simulink model "SPGF_FSK_0000_R2019b"  (R2019b)
settings: Solver=ode3  SolverName=ode4  StartTime=0.0  StopTime=1.4  FixedStep=50e-6/50  RelTol=1e-3  EnableMultiTasking=on
undefined symbols (not defined in the file): D11, Delta
libraries: powerlib x2544, powerlib_meascontrol x204, simulink x24
(part 32 of 33)

== system SPGF_FSK_0000_R2019b/W12/Q/breaker ==
  Fault A2 : Constant  Value=InitialStatus(3)
  Fault A3 : Constant  Value=InitialStatus(2)
  Fault A4 : Constant  Value=InitialStatus(1)
  Fault C1 : Constant  Value=SwitchC
  Fault C2 : Constant  Value=SwitchB
  Fault C3 : Constant  Value=SwitchA
  Ideal Switch A : powerlib/Power Electronics/Ideal Switch  Ron=BreakerResistance  Lon=0  IC=InitialStatus(1)  Rs=SnubberResistance  Cs=SnubberCapacitance  Measurements=off
  Ideal Switch B : powerlib/Power Electronics/Ideal Switch  Ron=BreakerResistance  Lon=0  IC=InitialStatus(2)  Rs=SnubberResistance  Cs=SnubberCapacitance  Measurements=off
  Ideal Switch C : powerlib/Power Electronics/Ideal Switch  Ron=BreakerResistance  Lon=0  IC=InitialStatus(3)  Rs=SnubberResistance  Cs=SnubberCapacitance  Measurements=off
  Stair Generator A : powerlib_meascontrol/Pulse & Signal Generators/Stair Generator  t=SwitchTimesA  e=SwitchStatusA  Ts=0
  Stair Generator B : powerlib_meascontrol/Pulse & Signal Generators/Stair Generator  t=SwitchTimesB  e=SwitchStatusB  Ts=0
  Stair Generator C : powerlib_meascontrol/Pulse & Signal Generators/Stair Generator  t=SwitchTimesB  e=SwitchStatusB  Ts=0
  Switch2 : Switch  Criteria=u2 > Threshold  Threshold=0.5
  Switch3 : Switch  Criteria=u2 > Threshold  Threshold=0.5
  Switch4 : Switch  Criteria=u2 > Threshold  Threshold=0.5
  A : PMIOPort  Side=Left
  B : PMIOPort  Port=2  Side=Left
  C : PMIOPort  Port=3  Side=Left
  a : PMIOPort  Port=4  Side=Right
  b : PMIOPort  Port=5  Side=Right
  c : PMIOPort  Port=6  Side=Right
  wires:
  Switch2/1 -> Ideal Switch C/1
  Fault A2/1 -> Switch2/3
  Fault C1/1 -> Switch2/2
  Switch3/1 -> Ideal Switch B/1
  Fault A3/1 -> Switch3/3
  Fault C2/1 -> Switch3/2
  Fault A4/1 -> Switch4/3
  Fault C3/1 -> Switch4/2
  Switch4/1 -> Ideal Switch A/1
  Stair Generator B/1 -> Switch3/1
  Stair Generator A/1 -> Switch4/1
  Stair Generator C/1 -> Switch2/1
  connections:
  Ideal Switch B/LConn1 -- B/RConn1
  Ideal Switch A/LConn1 -- A/RConn1
  Ideal Switch C/LConn1 -- C/RConn1
  Ideal Switch A/RConn1 -- a/RConn1
  b/RConn1 -- Ideal Switch B/RConn1
  c/RConn1 -- Ideal Switch C/RConn1

== system SPGF_FSK_0000_R2019b/W12/Q/meas ==
  Add : Sum  Inputs=+++
  GainI : Gain
  GainI0 : Gain
  I A: : powerlib/Measurements/Current Measurement  PhasorSimulation=off  OutputType=Complex  PSBequivalent=0
  I B: : powerlib/Measurements/Current Measurement  PhasorSimulation=off  OutputType=Complex  PSBequivalent=0
  I C: : powerlib/Measurements/Current Measurement  PhasorSimulation=off  OutputType=Complex  PSBequivalent=0
  Mux : Mux  Inputs=3
  A : PMIOPort  Side=Left
  B : PMIOPort  Port=2  Side=Left
  C : PMIOPort  Port=3  Side=Left
  a : PMIOPort  Port=4  Side=Right
  b : PMIOPort  Port=5  Side=Right
  c : PMIOPort  Port=6  Side=Right
  tag scope: CT3I0_W12=global, CTIabc_W12=global
  wires:
  I A:/1 -> Mux/1, Add/1
  I B:/1 -> Mux/2, Add/2
  I C:/1 -> Mux/3, Add/3
  Add/1 -> GainI0/1
  GainI0/1 -> [CT3I0_W12]
  Mux/1 -> GainI/1
  GainI/1 -> [CTIabc_W12]
  connections:
  I C:/RConn1 -- c/RConn1
  I B:/RConn1 -- b/RConn1
  a/RConn1 -- I A:/RConn1
  I A:/LConn1 -- A/RConn1
  I C:/LConn1 -- C/RConn1
  I B:/LConn1 -- B/RConn1

== system SPGF_FSK_0000_R2019b/W12/Q/shunt ==
  A : PMIOPort  Side=Left
  B : PMIOPort  Port=2  Side=Left
  C : PMIOPort  Port=3  Side=Left
  a : PMIOPort  Port=4  Side=Right
  b : PMIOPort  Port=5  Side=Right
  c : PMIOPort  Port=6  Side=Right
  connections:
  C/RConn1 -- c/RConn1
  B/RConn1 -- b/RConn1
  A/RConn1 -- a/RConn1

== system SPGF_FSK_0000_R2019b/W13/Q/breaker ==
  Fault A2 : Constant  Value=InitialStatus(3)
  Fault A3 : Constant  Value=InitialStatus(2)
  Fault A4 : Constant  Value=InitialStatus(1)
  Fault C1 : Constant  Value=SwitchC
  Fault C2 : Constant  Value=SwitchB
  Fault C3 : Constant  Value=SwitchA
  Ideal Switch A : powerlib/Power Electronics/Ideal Switch  Ron=BreakerResistance  Lon=0  IC=InitialStatus(1)  Rs=SnubberResistance  Cs=SnubberCapacitance  Measurements=off
  Ideal Switch B : powerlib/Power Electronics/Ideal Switch  Ron=BreakerResistance  Lon=0  IC=InitialStatus(2)  Rs=SnubberResistance  Cs=SnubberCapacitance  Measurements=off
  Ideal Switch C : powerlib/Power Electronics/Ideal Switch  Ron=BreakerResistance  Lon=0  IC=InitialStatus(3)  Rs=SnubberResistance  Cs=SnubberCapacitance  Measurements=off
  Stair Generator A : powerlib_meascontrol/Pulse & Signal Generators/Stair Generator  t=SwitchTimesA  e=SwitchStatusA  Ts=0
  Stair Generator B : powerlib_meascontrol/Pulse & Signal Generators/Stair Generator  t=SwitchTimesB  e=SwitchStatusB  Ts=0
  Stair Generator C : powerlib_meascontrol/Pulse & Signal Generators/Stair Generator  t=SwitchTimesB  e=SwitchStatusB  Ts=0
  Switch2 : Switch  Criteria=u2 > Threshold  Threshold=0.5
  Switch3 : Switch  Criteria=u2 > Threshold  Threshold=0.5
  Switch4 : Switch  Criteria=u2 > Threshold  Threshold=0.5
  A : PMIOPort  Side=Left
  B : PMIOPort  Port=2  Side=Left
  C : PMIOPort  Port=3  Side=Left
  a : PMIOPort  Port=4  Side=Right
  b : PMIOPort  Port=5  Side=Right
  c : PMIOPort  Port=6  Side=Right
  wires:
  Switch2/1 -> Ideal Switch C/1
  Fault A2/1 -> Switch2/3
  Fault C1/1 -> Switch2/2
  Switch3/1 -> Ideal Switch B/1
  Fault A3/1 -> Switch3/3
  Fault C2/1 -> Switch3/2
  Fault A4/1 -> Switch4/3
  Fault C3/1 -> Switch4/2
  Switch4/1 -> Ideal Switch A/1
  Stair Generator B/1 -> Switch3/1
  Stair Generator A/1 -> Switch4/1
  Stair Generator C/1 -> Switch2/1
  connections:
  Ideal Switch B/LConn1 -- B/RConn1
  Ideal Switch A/LConn1 -- A/RConn1
  Ideal Switch C/LConn1 -- C/RConn1
  Ideal Switch A/RConn1 -- a/RConn1
  b/RConn1 -- Ideal Switch B/RConn1
  c/RConn1 -- Ideal Switch C/RConn1

== system SPGF_FSK_0000_R2019b/W13/Q/meas ==
  Add : Sum  Inputs=+++
  GainI : Gain
  GainI0 : Gain
  I A: : powerlib/Measurements/Current Measurement  PhasorSimulation=off  OutputType=Complex  PSBequivalent=0
  I B: : powerlib/Measurements/Current Measurement  PhasorSimulation=off  OutputType=Complex  PSBequivalent=0
  I C: : powerlib/Measurements/Current Measurement  PhasorSimulation=off  OutputType=Complex  PSBequivalent=0
  Mux : Mux  Inputs=3
  A : PMIOPort  Side=Left
  B : PMIOPort  Port=2  Side=Left
  C : PMIOPort  Port=3  Side=Left
  a : PMIOPort  Port=4  Side=Right
  b : PMIOPort  Port=5  Side=Right
  c : PMIOPort  Port=6  Side=Right
  tag scope: CT3I0_W13=global, CTIabc_W13=global
  wires:
  I A:/1 -> Mux/1, Add/1
  I B:/1 -> Mux/2, Add/2
  I C:/1 -> Mux/3, Add/3
  Add/1 -> GainI0/1
  GainI0/1 -> [CT3I0_W13]
  Mux/1 -> GainI/1
  GainI/1 -> [CTIabc_W13]
  connections:
  I C:/RConn1 -- c/RConn1
  I B:/RConn1 -- b/RConn1
  a/RConn1 -- I A:/RConn1
  I A:/LConn1 -- A/RConn1
  I C:/LConn1 -- C/RConn1
  I B:/LConn1 -- B/RConn1

== system SPGF_FSK_0000_R2019b/W13/Q/shunt ==
  A : PMIOPort  Side=Left
  B : PMIOPort  Port=2  Side=Left
  C : PMIOPort  Port=3  Side=Left
  a : PMIOPort  Port=4  Side=Right
  b : PMIOPort  Port=5  Side=Right
  c : PMIOPort  Port=6  Side=Right
  connections:
  C/RConn1 -- c/RConn1
  B/RConn1 -- b/RConn1
  A/RConn1 -- a/RConn1

== system SPGF_FSK_0000_R2019b/W14/Q/breaker ==
  Fault A2 : Constant  Value=InitialStatus(3)
  Fault A3 : Constant  Value=InitialStatus(2)
  Fault A4 : Constant  Value=InitialStatus(1)
  Fault C1 : Constant  Value=SwitchC
  Fault C2 : Constant  Value=SwitchB
  Fault C3 : Constant  Value=SwitchA
  Ideal Switch A : powerlib/Power Electronics/Ideal Switch  Ron=BreakerResistance  Lon=0  IC=InitialStatus(1)  Rs=SnubberResistance  Cs=SnubberCapacitance  Measurements=off
  Ideal Switch B : powerlib/Power Electronics/Ideal Switch  Ron=BreakerResistance  Lon=0  IC=InitialStatus(2)  Rs=SnubberResistance  Cs=SnubberCapacitance  Measurements=off
  Ideal Switch C : powerlib/Power Electronics/Ideal Switch  Ron=BreakerResistance  Lon=0  IC=InitialStatus(3)  Rs=SnubberResistance  Cs=SnubberCapacitance  Measurements=off
  Stair Generator A : powerlib_meascontrol/Pulse & Signal Generators/Stair Generator  t=SwitchTimesA  e=SwitchStatusA  Ts=0
  Stair Generator B : powerlib_meascontrol/Pulse & Signal Generators/Stair Generator  t=SwitchTimesB  e=SwitchStatusB  Ts=0
  Stair Generator C : powerlib_meascontrol/Pulse & Signal Generators/Stair Generator  t=SwitchTimesB  e=SwitchStatusB  Ts=0
  Switch2 : Switch  Criteria=u2 > Threshold  Threshold=0.5
  Switch3 : Switch  Criteria=u2 > Threshold  Threshold=0.5
  Switch4 : Switch  Criteria=u2 > Threshold  Threshold=0.5
  A : PMIOPort  Side=Left
  B : PMIOPort  Port=2  Side=Left
  C : PMIOPort  Port=3  Side=Left
  a : PMIOPort  Port=4  Side=Right
  b : PMIOPort  Port=5  Side=Right
  c : PMIOPort  Port=6  Side=Right
  wires:
  Switch2/1 -> Ideal Switch C/1
  Fault A2/1 -> Switch2/3
  Fault C1/1 -> Switch2/2
  Switch3/1 -> Ideal Switch B/1
  Fault A3/1 -> Switch3/3
  Fault C2/1 -> Switch3/2
  Fault A4/1 -> Switch4/3
  Fault C3/1 -> Switch4/2
  Switch4/1 -> Ideal Switch A/1
  Stair Generator B/1 -> Switch3/1
  Stair Generator A/1 -> Switch4/1
  Stair Generator C/1 -> Switch2/1
  connections:
  Ideal Switch B/LConn1 -- B/RConn1
  Ideal Switch A/LConn1 -- A/RConn1
  Ideal Switch C/LConn1 -- C/RConn1
  Ideal Switch A/RConn1 -- a/RConn1
  b/RConn1 -- Ideal Switch B/RConn1
  c/RConn1 -- Ideal Switch C/RConn1

== system SPGF_FSK_0000_R2019b/W14/Q/meas ==
  Add : Sum  Inputs=+++
  GainI : Gain
  GainI0 : Gain
  I A: : powerlib/Measurements/Current Measurement  PhasorSimulation=off  OutputType=Complex  PSBequivalent=0
  I B: : powerlib/Measurements/Current Measurement  PhasorSimulation=off  OutputType=Complex  PSBequivalent=0
  I C: : powerlib/Measurements/Current Measurement  PhasorSimulation=off  OutputType=Complex  PSBequivalent=0
  Mux : Mux  Inputs=3
  A : PMIOPort  Side=Left
  B : PMIOPort  Port=2  Side=Left
  C : PMIOPort  Port=3  Side=Left
  a : PMIOPort  Port=4  Side=Right
  b : PMIOPort  Port=5  Side=Right
  c : PMIOPort  Port=6  Side=Right
  tag scope: CT3I0_W14=global, CTIabc_W14=global
  wires:
  I A:/1 -> Mux/1, Add/1
  I B:/1 -> Mux/2, Add/2
  I C:/1 -> Mux/3, Add/3
  Add/1 -> GainI0/1
  GainI0/1 -> [CT3I0_W14]
  Mux/1 -> GainI/1
  GainI/1 -> [CTIabc_W14]
  connections:
  I C:/RConn1 -- c/RConn1
  I B:/RConn1 -- b/RConn1
  a/RConn1 -- I A:/RConn1
  I A:/LConn1 -- A/RConn1
  I C:/LConn1 -- C/RConn1
  I B:/LConn1 -- B/RConn1

== system SPGF_FSK_0000_R2019b/W14/Q/shunt ==
  A : PMIOPort  Side=Left
  B : PMIOPort  Port=2  Side=Left
  C : PMIOPort  Port=3  Side=Left
  a : PMIOPort  Port=4  Side=Right
  b : PMIOPort  Port=5  Side=Right
  c : PMIOPort  Port=6  Side=Right
  connections:
  C/RConn1 -- c/RConn1
  B/RConn1 -- b/RConn1
  A/RConn1 -- a/RConn1

== system SPGF_FSK_0000_R2019b/W15/Q/breaker ==
  Fault A2 : Constant  Value=InitialStatus(3)
  Fault A3 : Constant  Value=InitialStatus(2)
  Fault A4 : Constant  Value=InitialStatus(1)
  Fault C1 : Constant  Value=SwitchC
  Fault C2 : Constant  Value=SwitchB
  Fault C3 : Constant  Value=SwitchA
  Ideal Switch A : powerlib/Power Electronics/Ideal Switch  Ron=BreakerResistance  Lon=0  IC=InitialStatus(1)  Rs=SnubberResistance  Cs=SnubberCapacitance  Measurements=off
  Ideal Switch B : powerlib/Power Electronics/Ideal Switch  Ron=BreakerResistance  Lon=0  IC=InitialStatus(2)  Rs=SnubberResistance  Cs=SnubberCapacitance  Measurements=off
  Ideal Switch C : powerlib/Power Electronics/Ideal Switch  Ron=BreakerResistance  Lon=0  IC=InitialStatus(3)  Rs=SnubberResistance  Cs=SnubberCapacitance  Measurements=off
  Stair Generator A : powerlib_meascontrol/Pulse & Signal Generators/Stair Generator  t=SwitchTimesA  e=SwitchStatusA  Ts=0
  Stair Generator B : powerlib_meascontrol/Pulse & Signal Generators/Stair Generator  t=SwitchTimesB  e=SwitchStatusB  Ts=0
  Stair Generator C : powerlib_meascontrol/Pulse & Signal Generators/Stair Generator  t=SwitchTimesB  e=SwitchStatusB  Ts=0
  Switch2 : Switch  Criteria=u2 > Threshold  Threshold=0.5
  Switch3 : Switch  Criteria=u2 > Threshold  Threshold=0.5
  Switch4 : Switch  Criteria=u2 > Threshold  Threshold=0.5
  A : PMIOPort  Side=Left
  B : PMIOPort  Port=2  Side=Left
  C : PMIOPort  Port=3  Side=Left
  a : PMIOPort  Port=4  Side=Right
  b : PMIOPort  Port=5  Side=Right
  c : PMIOPort  Port=6  Side=Right
  wires:
  Switch2/1 -> Ideal Switch C/1
  Fault A2/1 -> Switch2/3
  Fault C1/1 -> Switch2/2
  Switch3/1 -> Ideal Switch B/1
  Fault A3/1 -> Switch3/3
  Fault C2/1 -> Switch3/2
  Fault A4/1 -> Switch4/3
  Fault C3/1 -> Switch4/2
  Switch4/1 -> Ideal Switch A/1
  Stair Generator B/1 -> Switch3/1
  Stair Generator A/1 -> Switch4/1
  Stair Generator C/1 -> Switch2/1
  connections:
  Ideal Switch B/LConn1 -- B/RConn1
  Ideal Switch A/LConn1 -- A/RConn1
  Ideal Switch C/LConn1 -- C/RConn1
  Ideal Switch A/RConn1 -- a/RConn1
  b/RConn1 -- Ideal Switch B/RConn1
  c/RConn1 -- Ideal Switch C/RConn1

== system SPGF_FSK_0000_R2019b/W15/Q/meas ==
  Add : Sum  Inputs=+++
  GainI : Gain
  GainI0 : Gain
  I A: : powerlib/Measurements/Current Measurement  PhasorSimulation=off  OutputType=Complex  PSBequivalent=0
  I B: : powerlib/Measurements/Current Measurement  PhasorSimulation=off  OutputType=Complex  PSBequivalent=0
  I C: : powerlib/Measurements/Current Measurement  PhasorSimulation=off  OutputType=Complex  PSBequivalent=0
  Mux : Mux  Inputs=3
  A : PMIOPort  Side=Left
  B : PMIOPort  Port=2  Side=Left
  C : PMIOPort  Port=3  Side=Left
  a : PMIOPort  Port=4  Side=Right
  b : PMIOPort  Port=5  Side=Right
  c : PMIOPort  Port=6  Side=Right
  tag scope: CT3I0_W15=global, CTIabc_W15=global
  wires:
  I A:/1 -> Mux/1, Add/1
  I B:/1 -> Mux/2, Add/2
  I C:/1 -> Mux/3, Add/3
  Add/1 -> GainI0/1
  GainI0/1 -> [CT3I0_W15]
  Mux/1 -> GainI/1
  GainI/1 -> [CTIabc_W15]
  connections:
  I C:/RConn1 -- c/RConn1
  I B:/RConn1 -- b/RConn1
  a/RConn1 -- I A:/RConn1
  I A:/LConn1 -- A/RConn1
  I C:/LConn1 -- C/RConn1
  I B:/LConn1 -- B/RConn1

== system SPGF_FSK_0000_R2019b/W15/Q/shunt ==
  A : PMIOPort  Side=Left
  B : PMIOPort  Port=2  Side=Left
  C : PMIOPort  Port=3  Side=Left
  a : PMIOPort  Port=4  Side=Right
  b : PMIOPort  Port=5  Side=Right
  c : PMIOPort  Port=6  Side=Right
  connections:
  C/RConn1 -- c/RConn1
  B/RConn1 -- b/RConn1
  A/RConn1 -- a/RConn1

== system SPGF_FSK_0000_R2019b/W21/Q/breaker ==
  Fault A2 : Constant  Value=InitialStatus(3)
  Fault A3 : Constant  Value=InitialStatus(2)
  Fault A4 : Constant  Value=InitialStatus(1)
  Fault C1 : Constant  Value=SwitchC
  Fault C2 : Constant  Value=SwitchB
  Fault C3 : Constant  Value=SwitchA
  Ideal Switch A : powerlib/Power Electronics/Ideal Switch  Ron=BreakerResistance  Lon=0  IC=InitialStatus(1)  Rs=SnubberResistance  Cs=SnubberCapacitance  Measurements=off
  Ideal Switch B : powerlib/Power Electronics/Ideal Switch  Ron=BreakerResistance  Lon=0  IC=InitialStatus(2)  Rs=SnubberResistance  Cs=SnubberCapacitance  Measurements=off
  Ideal Switch C : powerlib/Power Electronics/Ideal Switch  Ron=BreakerResistance  Lon=0  IC=InitialStatus(3)  Rs=SnubberResistance  Cs=SnubberCapacitance  Measurements=off
  Stair Generator A : powerlib_meascontrol/Pulse & Signal Generators/Stair Generator  t=SwitchTimesA  e=SwitchStatusA  Ts=0
  Stair Generator B : powerlib_meascontrol/Pulse & Signal Generators/Stair Generator  t=SwitchTimesB  e=SwitchStatusB  Ts=0
  Stair Generator C : powerlib_meascontrol/Pulse & Signal Generators/Stair Generator  t=SwitchTimesC  e=SwitchStatusC  Ts=0
  Switch2 : Switch  Criteria=u2 > Threshold  Threshold=0.5
  Switch3 : Switch  Criteria=u2 > Threshold  Threshold=0.5
  Switch4 : Switch  Criteria=u2 > Threshold  Threshold=0.5
  A : PMIOPort  Side=Left
  B : PMIOPort  Port=2  Side=Left
  C : PMIOPort  Port=3  Side=Left
  a : PMIOPort  Port=4  Side=Right
  b : PMIOPort  Port=5  Side=Right
  c : PMIOPort  Port=6  Side=Right
  wires:
  Switch2/1 -> Ideal Switch C/1
  Fault A2/1 -> Switch2/3
  Fault C1/1 -> Switch2/2
  Switch3/1 -> Ideal Switch B/1
  Fault A3/1 -> Switch3/3
  Fault C2/1 -> Switch3/2
  Fault A4/1 -> Switch4/3
  Fault C3/1 -> Switch4/2
  Switch4/1 -> Ideal Switch A/1
  Stair Generator B/1 -> Switch3/1
  Stair Generator A/1 -> Switch4/1
  Stair Generator C/1 -> Switch2/1
  connections:
  Ideal Switch B/LConn1 -- B/RConn1
  Ideal Switch A/LConn1 -- A/RConn1
  Ideal Switch C/LConn1 -- C/RConn1
  Ideal Switch A/RConn1 -- a/RConn1
  b/RConn1 -- Ideal Switch B/RConn1
  c/RConn1 -- Ideal Switch C/RConn1

== system SPGF_FSK_0000_R2019b/W21/Q/meas ==
  Add : Sum  Inputs=+++
  GainI : Gain
  GainI0 : Gain
  I A: : powerlib/Measurements/Current Measurement  PhasorSimulation=off  OutputType=Complex  PSBequivalent=0
  I B: : powerlib/Measurements/Current Measurement  PhasorSimulation=off  OutputType=Complex  PSBequivalent=0
  I C: : powerlib/Measurements/Current Measurement  PhasorSimulation=off  OutputType=Complex  PSBequivalent=0
  Mux : Mux  Inputs=3
  A : PMIOPort  Side=Left
  B : PMIOPort  Port=2  Side=Left
  C : PMIOPort  Port=3  Side=Left
  a : PMIOPort  Port=4  Side=Right
  b : PMIOPort  Port=5  Side=Right
  c : PMIOPort  Port=6  Side=Right
  tag scope: CT3I0_W21=global, CTIabc_W21=global
  wires:
  I A:/1 -> Mux/1, Add/1
  I B:/1 -> Mux/2, Add/2
  I C:/1 -> Mux/3, Add/3
  Add/1 -> GainI0/1
  GainI0/1 -> [CT3I0_W21]
  Mux/1 -> GainI/1
  GainI/1 -> [CTIabc_W21]
  connections:
  I C:/RConn1 -- c/RConn1
  I B:/RConn1 -- b/RConn1
  a/RConn1 -- I A:/RConn1
  I A:/LConn1 -- A/RConn1
  I C:/LConn1 -- C/RConn1
  I B:/LConn1 -- B/RConn1

== system SPGF_FSK_0000_R2019b/W21/Q/shunt ==
  A : PMIOPort  Side=Left
  B : PMIOPort  Port=2  Side=Left
  C : PMIOPort  Port=3  Side=Left
  a : PMIOPort  Port=4  Side=Right
  b : PMIOPort  Port=5  Side=Right
  c : PMIOPort  Port=6  Side=Right
  connections:
  C/RConn1 -- c/RConn1
  B/RConn1 -- b/RConn1
  A/RConn1 -- a/RConn1

== system SPGF_FSK_0000_R2019b/W22/Q/breaker ==
  Fault A2 : Constant  Value=InitialStatus(3)
  Fault A3 : Constant  Value=InitialStatus(2)
  Fault A4 : Constant  Value=InitialStatus(1)
  Fault C1 : Constant  Value=SwitchC
  Fault C2 : Constant  Value=SwitchB
  Fault C3 : Constant  Value=SwitchA
  Ideal Switch A : powerlib/Power Electronics/Ideal Switch  Ron=BreakerResistance  Lon=0  IC=InitialStatus(1)  Rs=SnubberResistance  Cs=SnubberCapacitance  Measurements=off
  Ideal Switch B : powerlib/Power Electronics/Ideal Switch  Ron=BreakerResistance  Lon=0  IC=InitialStatus(2)  Rs=SnubberResistance  Cs=SnubberCapacitance  Measurements=off
  Ideal Switch C : powerlib/Power Electronics/Ideal Switch  Ron=BreakerResistance  Lon=0  IC=InitialStatus(3)  Rs=SnubberResistance  Cs=SnubberCapacitance  Measurements=off
  Stair Generator A : powerlib_meascontrol/Pulse & Signal Generators/Stair Generator  t=SwitchTimesA  e=SwitchStatusA  Ts=0
  Stair Generator B : powerlib_meascontrol/Pulse & Signal Generators/Stair Generator  t=SwitchTimesB  e=SwitchStatusB  Ts=0
  Stair Generator C : powerlib_meascontrol/Pulse & Signal Generators/Stair Generator  t=SwitchTimesB  e=SwitchStatusB  Ts=0
  Switch2 : Switch  Criteria=u2 > Threshold  Threshold=0.5
  Switch3 : Switch  Criteria=u2 > Threshold  Threshold=0.5
  Switch4 : Switch  Criteria=u2 > Threshold  Threshold=0.5
  A : PMIOPort  Side=Left
  B : PMIOPort  Port=2  Side=Left
  C : PMIOPort  Port=3  Side=Left
  a : PMIOPort  Port=4  Side=Right
  b : PMIOPort  Port=5  Side=Right
  c : PMIOPort  Port=6  Side=Right
  wires:
  Switch2/1 -> Ideal Switch C/1
  Fault A2/1 -> Switch2/3
  Fault C1/1 -> Switch2/2
  Switch3/1 -> Ideal Switch B/1
  Fault A3/1 -> Switch3/3
  Fault C2/1 -> Switch3/2
  Fault A4/1 -> Switch4/3
  Fault C3/1 -> Switch4/2
  Switch4/1 -> Ideal Switch A/1
  Stair Generator B/1 -> Switch3/1
  Stair Generator A/1 -> Switch4/1
  Stair Generator C/1 -> Switch2/1
  connections:
  Ideal Switch B/LConn1 -- B/RConn1
  Ideal Switch A/LConn1 -- A/RConn1
  Ideal Switch C/LConn1 -- C/RConn1
  Ideal Switch A/RConn1 -- a/RConn1
  b/RConn1 -- Ideal Switch B/RConn1
  c/RConn1 -- Ideal Switch C/RConn1

== system SPGF_FSK_0000_R2019b/W22/Q/meas ==
  Add : Sum  Inputs=+++
  GainI : Gain
  GainI0 : Gain
  I A: : powerlib/Measurements/Current Measurement  PhasorSimulation=off  OutputType=Complex  PSBequivalent=0
  I B: : powerlib/Measurements/Current Measurement  PhasorSimulation=off  OutputType=Complex  PSBequivalent=0
  I C: : powerlib/Measurements/Current Measurement  PhasorSimulation=off  OutputType=Complex  PSBequivalent=0
  Mux : Mux  Inputs=3
  A : PMIOPort  Side=Left
  B : PMIOPort  Port=2  Side=Left
  C : PMIOPort  Port=3  Side=Left
  a : PMIOPort  Port=4  Side=Right
  b : PMIOPort  Port=5  Side=Right
  c : PMIOPort  Port=6  Side=Right
  tag scope: CT3I0_W22=global, CTIabc_W22=global
  wires:
  I A:/1 -> Mux/1, Add/1
  I B:/1 -> Mux/2, Add/2
  I C:/1 -> Mux/3, Add/3
  Add/1 -> GainI0/1
  GainI0/1 -> [CT3I0_W22]
  Mux/1 -> GainI/1
  GainI/1 -> [CTIabc_W22]
  connections:
  I C:/RConn1 -- c/RConn1
  I B:/RConn1 -- b/RConn1
  a/RConn1 -- I A:/RConn1
  I A:/LConn1 -- A/RConn1
  I C:/LConn1 -- C/RConn1
  I B:/LConn1 -- B/RConn1

== system SPGF_FSK_0000_R2019b/W22/Q/shunt ==
  A : PMIOPort  Side=Left
  B : PMIOPort  Port=2  Side=Left
  C : PMIOPort  Port=3  Side=Left
  a : PMIOPort  Port=4  Side=Right
  b : PMIOPort  Port=5  Side=Right
  c : PMIOPort  Port=6  Side=Right
  connections:
  C/RConn1 -- c/RConn1
  B/RConn1 -- b/RConn1
  A/RConn1 -- a/RConn1

== system SPGF_FSK_0000_R2019b/W31/Q/breaker ==
  Fault A2 : Constant  Value=InitialStatus(3)
  Fault A3 : Constant  Value=InitialStatus(2)
  Fault A4 : Constant  Value=InitialStatus(1)
  Fault C1 : Constant  Value=SwitchC
  Fault C2 : Constant  Value=SwitchB
  Fault C3 : Constant  Value=SwitchA
  Ideal Switch A : powerlib/Power Electronics/Ideal Switch  Ron=BreakerResistance  Lon=0  IC=InitialStatus(1)  Rs=SnubberResistance  Cs=SnubberCapacitance  Measurements=off
  Ideal Switch B : powerlib/Power Electronics/Ideal Switch  Ron=BreakerResistance  Lon=0  IC=InitialStatus(2)  Rs=SnubberResistance  Cs=SnubberCapacitance  Measurements=off
  Ideal Switch C : powerlib/Power Electronics/Ideal Switch  Ron=BreakerResistance  Lon=0  IC=InitialStatus(3)  Rs=SnubberResistance  Cs=SnubberCapacitance  Measurements=off
  Stair Generator A : powerlib_meascontrol/Pulse & Signal Generators/Stair Generator  t=SwitchTimesA  e=SwitchStatusA  Ts=0
  Stair Generator B : powerlib_meascontrol/Pulse & Signal Generators/Stair Generator  t=SwitchTimesB  e=SwitchStatusB  Ts=0
  Stair Generator C : powerlib_meascontrol/Pulse & Signal Generators/Stair Generator  t=SwitchTimesC  e=SwitchStatusC  Ts=0
  Switch2 : Switch  Criteria=u2 > Threshold  Threshold=0.5
  Switch3 : Switch  Criteria=u2 > Threshold  Threshold=0.5
  Switch4 : Switch  Criteria=u2 > Threshold  Threshold=0.5
  A : PMIOPort  Side=Left
  B : PMIOPort  Port=2  Side=Left
  C : PMIOPort  Port=3  Side=Left
  a : PMIOPort  Port=4  Side=Right
  b : PMIOPort  Port=5  Side=Right
  c : PMIOPort  Port=6  Side=Right
  wires:
  Switch2/1 -> Ideal Switch C/1
  Fault A2/1 -> Switch2/3
  Fault C1/1 -> Switch2/2
  Switch3/1 -> Ideal Switch B/1
  Fault A3/1 -> Switch3/3
  Fault C2/1 -> Switch3/2
  Fault A4/1 -> Switch4/3
  Fault C3/1 -> Switch4/2
  Switch4/1 -> Ideal Switch A/1
  Stair Generator B/1 -> Switch3/1
  Stair Generator A/1 -> Switch4/1
  Stair Generator C/1 -> Switch2/1
  connections:
  Ideal Switch B/LConn1 -- B/RConn1
  Ideal Switch A/LConn1 -- A/RConn1
  Ideal Switch C/LConn1 -- C/RConn1
  Ideal Switch A/RConn1 -- a/RConn1
  b/RConn1 -- Ideal Switch B/RConn1
  c/RConn1 -- Ideal Switch C/RConn1

== system SPGF_FSK_0000_R2019b/W31/Q/meas ==
  Add : Sum  Inputs=+++
  GainI : Gain
  GainI0 : Gain
  I A: : powerlib/Measurements/Current Measurement  PhasorSimulation=off  OutputType=Complex  PSBequivalent=0
  I B: : powerlib/Measurements/Current Measurement  PhasorSimulation=off  OutputType=Complex  PSBequivalent=0
  I C: : powerlib/Measurements/Current Measurement  PhasorSimulation=off  OutputType=Complex  PSBequivalent=0
  Mux : Mux  Inputs=3
  A : PMIOPort  Side=Left
  B : PMIOPort  Port=2  Side=Left
  C : PMIOPort  Port=3  Side=Left
  a : PMIOPort  Port=4  Side=Right
  b : PMIOPort  Port=5  Side=Right
  c : PMIOPort  Port=6  Side=Right
  tag scope: CT3I0_W31=global, CTIabc_W31=global
  wires:
  I A:/1 -> Mux/1, Add/1
  I B:/1 -> Mux/2, Add/2
  I C:/1 -> Mux/3, Add/3
  Add/1 -> GainI0/1
  GainI0/1 -> [CT3I0_W31]
  Mux/1 -> GainI/1
  GainI/1 -> [CTIabc_W31]
  connections:
  I C:/RConn1 -- c/RConn1
  I B:/RConn1 -- b/RConn1
  a/RConn1 -- I A:/RConn1
  I A:/LConn1 -- A/RConn1
  I C:/LConn1 -- C/RConn1
  I B:/LConn1 -- B/RConn1

== system SPGF_FSK_0000_R2019b/W31/Q/shunt ==
  A : PMIOPort  Side=Left
  B : PMIOPort  Port=2  Side=Left
  C : PMIOPort  Port=3  Side=Left
  a : PMIOPort  Port=4  Side=Right
  b : PMIOPort  Port=5  Side=Right
  c : PMIOPort  Port=6  Side=Right
  connections:
  C/RConn1 -- c/RConn1
  B/RConn1 -- b/RConn1
  A/RConn1 -- a/RConn1

== system SPGF_FSK_0000_R2019b/W32/Q/breaker ==
  Fault A2 : Constant  Value=InitialStatus(3)
  Fault A3 : Constant  Value=InitialStatus(2)
  Fault A4 : Constant  Value=InitialStatus(1)
  Fault C1 : Constant  Value=SwitchC
  Fault C2 : Constant  Value=SwitchB
  Fault C3 : Constant  Value=SwitchA
  Ideal Switch A : powerlib/Power Electronics/Ideal Switch  Ron=BreakerResistance  Lon=0  IC=InitialStatus(1)  Rs=SnubberResistance  Cs=SnubberCapacitance  Measurements=off
  Ideal Switch B : powerlib/Power Electronics/Ideal Switch  Ron=BreakerResistance  Lon=0  IC=InitialStatus(2)  Rs=SnubberResistance  Cs=SnubberCapacitance  Measurements=off
  Ideal Switch C : powerlib/Power Electronics/Ideal Switch  Ron=BreakerResistance  Lon=0  IC=InitialStatus(3)  Rs=SnubberResistance  Cs=SnubberCapacitance  Measurements=off
  Stair Generator A : powerlib_meascontrol/Pulse & Signal Generators/Stair Generator  t=SwitchTimesA  e=SwitchStatusA  Ts=0
  Stair Generator B : powerlib_meascontrol/Pulse & Signal Generators/Stair Generator  t=SwitchTimesB  e=SwitchStatusB  Ts=0
  Stair Generator C : powerlib_meascontrol/Pulse & Signal Generators/Stair Generator  t=SwitchTimesB  e=SwitchStatusB  Ts=0
  Switch2 : Switch  Criteria=u2 > Threshold  Threshold=0.5
  Switch3 : Switch  Criteria=u2 > Threshold  Threshold=0.5
  Switch4 : Switch  Criteria=u2 > Threshold  Threshold=0.5
  A : PMIOPort  Side=Left
  B : PMIOPort  Port=2  Side=Left
  C : PMIOPort  Port=3  Side=Left
  a : PMIOPort  Port=4  Side=Right
  b : PMIOPort  Port=5  Side=Right
  c : PMIOPort  Port=6  Side=Right
  wires:
  Switch2/1 -> Ideal Switch C/1
  Fault A2/1 -> Switch2/3
  Fault C1/1 -> Switch2/2
  Switch3/1 -> Ideal Switch B/1
  Fault A3/1 -> Switch3/3
  Fault C2/1 -> Switch3/2
  Fault A4/1 -> Switch4/3
  Fault C3/1 -> Switch4/2
  Switch4/1 -> Ideal Switch A/1
  Stair Generator B/1 -> Switch3/1
  Stair Generator A/1 -> Switch4/1
  Stair Generator C/1 -> Switch2/1
  connections:
  Ideal Switch B/LConn1 -- B/RConn1
  Ideal Switch A/LConn1 -- A/RConn1
  Ideal Switch C/LConn1 -- C/RConn1
  Ideal Switch A/RConn1 -- a/RConn1
  b/RConn1 -- Ideal Switch B/RConn1
  c/RConn1 -- Ideal Switch C/RConn1

== system SPGF_FSK_0000_R2019b/W32/Q/meas ==
  Add : Sum  Inputs=+++
  GainI : Gain
  GainI0 : Gain
  I A: : powerlib/Measurements/Current Measurement  PhasorSimulation=off  OutputType=Complex  PSBequivalent=0
  I B: : powerlib/Measurements/Current Measurement  PhasorSimulation=off  OutputType=Complex  PSBequivalent=0
  I C: : powerlib/Measurements/Current Measurement  PhasorSimulation=off  OutputType=Complex  PSBequivalent=0
  Mux : Mux  Inputs=3
  A : PMIOPort  Side=Left
  B : PMIOPort  Port=2  Side=Left
  C : PMIOPort  Port=3  Side=Left
  a : PMIOPort  Port=4  Side=Right
  b : PMIOPort  Port=5  Side=Right
  c : PMIOPort  Port=6  Side=Right
  tag scope: CT3I0_W32=global, CTIabc_W32=global
  wires:
  I A:/1 -> Mux/1, Add/1
  I B:/1 -> Mux/2, Add/2
  I C:/1 -> Mux/3, Add/3
  Add/1 -> GainI0/1
  GainI0/1 -> [CT3I0_W32]
  Mux/1 -> GainI/1
  GainI/1 -> [CTIabc_W32]
  connections:
  I C:/RConn1 -- c/RConn1
  I B:/RConn1 -- b/RConn1
  a/RConn1 -- I A:/RConn1
  I A:/LConn1 -- A/RConn1
  I C:/LConn1 -- C/RConn1
  I B:/LConn1 -- B/RConn1

== system SPGF_FSK_0000_R2019b/W32/Q/shunt ==
  A : PMIOPort  Side=Left
  B : PMIOPort  Port=2  Side=Left
  C : PMIOPort  Port=3  Side=Left
  a : PMIOPort  Port=4  Side=Right
  b : PMIOPort  Port=5  Side=Right
  c : PMIOPort  Port=6  Side=Right
  connections:
  C/RConn1 -- c/RConn1
  B/RConn1 -- b/RConn1
  A/RConn1 -- a/RConn1

== system SPGF_FSK_0000_R2019b/W33/Q/breaker ==
  Fault A2 : Constant  Value=InitialStatus(3)
  Fault A3 : Constant  Value=InitialStatus(2)
  Fault A4 : Constant  Value=InitialStatus(1)
  Fault C1 : Constant  Value=SwitchC
  Fault C2 : Constant  Value=SwitchB
  Fault C3 : Constant  Value=SwitchA
  Ideal Switch A : powerlib/Power Electronics/Ideal Switch  Ron=BreakerResistance  Lon=0  IC=InitialStatus(1)  Rs=SnubberResistance  Cs=SnubberCapacitance  Measurements=off
  Ideal Switch B : powerlib/Power Electronics/Ideal Switch  Ron=BreakerResistance  Lon=0  IC=InitialStatus(2)  Rs=SnubberResistance  Cs=SnubberCapacitance  Measurements=off
  Ideal Switch C : powerlib/Power Electronics/Ideal Switch  Ron=BreakerResistance  Lon=0  IC=InitialStatus(3)  Rs=SnubberResistance  Cs=SnubberCapacitance  Measurements=off
  Stair Generator A : powerlib_meascontrol/Pulse & Signal Generators/Stair Generator  t=SwitchTimesA  e=SwitchStatusA  Ts=0
  Stair Generator B : powerlib_meascontrol/Pulse & Signal Generators/Stair Generator  t=SwitchTimesB  e=SwitchStatusB  Ts=0
  Stair Generator C : powerlib_meascontrol/Pulse & Signal Generators/Stair Generator  t=SwitchTimesB  e=SwitchStatusB  Ts=0
  Switch2 : Switch  Criteria=u2 > Threshold  Threshold=0.5
  Switch3 : Switch  Criteria=u2 > Threshold  Threshold=0.5
  Switch4 : Switch  Criteria=u2 > Threshold  Threshold=0.5
  A : PMIOPort  Side=Left
  B : PMIOPort  Port=2  Side=Left
  C : PMIOPort  Port=3  Side=Left
  a : PMIOPort  Port=4  Side=Right
  b : PMIOPort  Port=5  Side=Right
  c : PMIOPort  Port=6  Side=Right
  wires:
  Switch2/1 -> Ideal Switch C/1
  Fault A2/1 -> Switch2/3
  Fault C1/1 -> Switch2/2
  Switch3/1 -> Ideal Switch B/1
  Fault A3/1 -> Switch3/3
  Fault C2/1 -> Switch3/2
  Fault A4/1 -> Switch4/3
  Fault C3/1 -> Switch4/2
  Switch4/1 -> Ideal Switch A/1
  Stair Generator B/1 -> Switch3/1
  Stair Generator A/1 -> Switch4/1
  Stair Generator C/1 -> Switch2/1
  connections:
  Ideal Switch B/LConn1 -- B/RConn1
  Ideal Switch A/LConn1 -- A/RConn1
  Ideal Switch C/LConn1 -- C/RConn1
  Ideal Switch A/RConn1 -- a/RConn1
  b/RConn1 -- Ideal Switch B/RConn1
  c/RConn1 -- Ideal Switch C/RConn1

== system SPGF_FSK_0000_R2019b/W33/Q/meas ==
  Add : Sum  Inputs=+++
  GainI : Gain
  GainI0 : Gain
  I A: : powerlib/Measurements/Current Measurement  PhasorSimulation=off  OutputType=Complex  PSBequivalent=0
  I B: : powerlib/Measurements/Current Measurement  PhasorSimulation=off  OutputType=Complex  PSBequivalent=0
  I C: : powerlib/Measurements/Current Measurement  PhasorSimulation=off  OutputType=Complex  PSBequivalent=0
  Mux : Mux  Inputs=3
  A : PMIOPort  Side=Left
  B : PMIOPort  Port=2  Side=Left
  C : PMIOPort  Port=3  Side=Left
  a : PMIOPort  Port=4  Side=Right
  b : PMIOPort  Port=5  Side=Right
  c : PMIOPort  Port=6  Side=Right
  tag scope: CT3I0_W33=global, CTIabc_W33=global
  wires:
  I A:/1 -> Mux/1, Add/1
  I B:/1 -> Mux/2, Add/2
  I C:/1 -> Mux/3, Add/3
  Add/1 -> GainI0/1
  GainI0/1 -> [CT3I0_W33]
  Mux/1 -> GainI/1
  GainI/1 -> [CTIabc_W33]
  connections:
  I C:/RConn1 -- c/RConn1
  I B:/RConn1 -- b/RConn1
  a/RConn1 -- I A:/RConn1
  I A:/LConn1 -- A/RConn1
  I C:/LConn1 -- C/RConn1
  I B:/LConn1 -- B/RConn1

== system SPGF_FSK_0000_R2019b/W33/Q/shunt ==
  A : PMIOPort  Side=Left
  B : PMIOPort  Port=2  Side=Left
  C : PMIOPort  Port=3  Side=Left
  a : PMIOPort  Port=4  Side=Right
  b : PMIOPort  Port=5  Side=Right
  c : PMIOPort  Port=6  Side=Right
  connections:
  C/RConn1 -- c/RConn1
  B/RConn1 -- b/RConn1
  A/RConn1 -- a/RConn1

== system SPGF_FSK_0000_R2019b/W34/Q/breaker ==
  Fault A2 : Constant  Value=InitialStatus(3)
  Fault A3 : Constant  Value=InitialStatus(2)
  Fault A4 : Constant  Value=InitialStatus(1)
  Fault C1 : Constant  Value=SwitchC
  Fault C2 : Constant  Value=SwitchB
  Fault C3 : Constant  Value=SwitchA
  Ideal Switch A : powerlib/Power Electronics/Ideal Switch  Ron=BreakerResistance  Lon=0  IC=InitialStatus(1)  Rs=SnubberResistance  Cs=SnubberCapacitance  Measurements=off
  Ideal Switch B : powerlib/Power Electronics/Ideal Switch  Ron=BreakerResistance  Lon=0  IC=InitialStatus(2)  Rs=SnubberResistance  Cs=SnubberCapacitance  Measurements=off
  Ideal Switch C : powerlib/Power Electronics/Ideal Switch  Ron=BreakerResistance  Lon=0  IC=InitialStatus(3)  Rs=SnubberResistance  Cs=SnubberCapacitance  Measurements=off
  Stair Generator A : powerlib_meascontrol/Pulse & Signal Generators/Stair Generator  t=SwitchTimesA  e=SwitchStatusA  Ts=0
  Stair Generator B : powerlib_meascontrol/Pulse & Signal Generators/Stair Generator  t=SwitchTimesB  e=SwitchStatusB  Ts=0
  Stair Generator C : powerlib_meascontrol/Pulse & Signal Generators/Stair Generator  t=SwitchTimesB  e=SwitchStatusB  Ts=0
  Switch2 : Switch  Criteria=u2 > Threshold  Threshold=0.5
  Switch3 : Switch  Criteria=u2 > Threshold  Threshold=0.5
  Switch4 : Switch  Criteria=u2 > Threshold  Threshold=0.5
  A : PMIOPort  Side=Left
  B : PMIOPort  Port=2  Side=Left
  C : PMIOPort  Port=3  Side=Left
  a : PMIOPort  Port=4  Side=Right
  b : PMIOPort  Port=5  Side=Right
  c : PMIOPort  Port=6  Side=Right
  wires:
  Switch2/1 -> Ideal Switch C/1
  Fault A2/1 -> Switch2/3
  Fault C1/1 -> Switch2/2
  Switch3/1 -> Ideal Switch B/1
  Fault A3/1 -> Switch3/3
  Fault C2/1 -> Switch3/2
  Fault A4/1 -> Switch4/3
  Fault C3/1 -> Switch4/2
  Switch4/1 -> Ideal Switch A/1
  Stair Generator B/1 -> Switch3/1
  Stair Generator A/1 -> Switch4/1
  Stair Generator C/1 -> Switch2/1
  connections:
  Ideal Switch B/LConn1 -- B/RConn1
  Ideal Switch A/LConn1 -- A/RConn1
  Ideal Switch C/LConn1 -- C/RConn1
  Ideal Switch A/RConn1 -- a/RConn1
  b/RConn1 -- Ideal Switch B/RConn1
  c/RConn1 -- Ideal Switch C/RConn1

== system SPGF_FSK_0000_R2019b/W34/Q/meas ==
  Add : Sum  Inputs=+++
  GainI : Gain
  GainI0 : Gain
  I A: : powerlib/Measurements/Current Measurement  PhasorSimulation=off  OutputType=Complex  PSBequivalent=0
  I B: : powerlib/Measurements/Current Measurement  PhasorSimulation=off  OutputType=Complex  PSBequivalent=0
  I C: : powerlib/Measurements/Current Measurement  PhasorSimulation=off  OutputType=Complex  PSBequivalent=0
  Mux : Mux  Inputs=3
  A : PMIOPort  Side=Left
  B : PMIOPort  Port=2  Side=Left
  C : PMIOPort  Port=3  Side=Left
  a : PMIOPort  Port=4  Side=Right
  b : PMIOPort  Port=5  Side=Right
  c : PMIOPort  Port=6  Side=Right
  tag scope: CT3I0_W34=global, CTIabc_W34=global
  wires:
  I A:/1 -> Mux/1, Add/1
  I B:/1 -> Mux/2, Add/2
  I C:/1 -> Mux/3, Add/3
  Add/1 -> GainI0/1
  GainI0/1 -> [CT3I0_W34]
  Mux/1 -> GainI/1
  GainI/1 -> [CTIabc_W34]
  connections:
  I C:/RConn1 -- c/RConn1
  I B:/RConn1 -- b/RConn1
  a/RConn1 -- I A:/RConn1
  I A:/LConn1 -- A/RConn1
  I C:/LConn1 -- C/RConn1
  I B:/LConn1 -- B/RConn1

== system SPGF_FSK_0000_R2019b/W34/Q/shunt ==
  A : PMIOPort  Side=Left
  B : PMIOPort  Port=2  Side=Left
  C : PMIOPort  Port=3  Side=Left
  a : PMIOPort  Port=4  Side=Right
  b : PMIOPort  Port=5  Side=Right
  c : PMIOPort  Port=6  Side=Right
  connections:
  C/RConn1 -- c/RConn1
  B/RConn1 -- b/RConn1
  A/RConn1 -- a/RConn1

== system SPGF_FSK_0000_R2019b/W35/Q/breaker ==
  Fault A2 : Constant  Value=InitialStatus(3)
  Fault A3 : Constant  Value=InitialStatus(2)
  Fault A4 : Constant  Value=InitialStatus(1)
  Fault C1 : Constant  Value=SwitchC
  Fault C2 : Constant  Value=SwitchB
  Fault C3 : Constant  Value=SwitchA
  Ideal Switch A : powerlib/Power Electronics/Ideal Switch  Ron=BreakerResistance  Lon=0  IC=InitialStatus(1)  Rs=SnubberResistance  Cs=SnubberCapacitance  Measurements=off
  Ideal Switch B : powerlib/Power Electronics/Ideal Switch  Ron=BreakerResistance  Lon=0  IC=InitialStatus(2)  Rs=SnubberResistance  Cs=SnubberCapacitance  Measurements=off
  Ideal Switch C : powerlib/Power Electronics/Ideal Switch  Ron=BreakerResistance  Lon=0  IC=InitialStatus(3)  Rs=SnubberResistance  Cs=SnubberCapacitance  Measurements=off
  Stair Generator A : powerlib_meascontrol/Pulse & Signal Generators/Stair Generator  t=SwitchTimesA  e=SwitchStatusA  Ts=0
  Stair Generator B : powerlib_meascontrol/Pulse & Signal Generators/Stair Generator  t=SwitchTimesB  e=SwitchStatusB  Ts=0
  Stair Generator C : powerlib_meascontrol/Pulse & Signal Generators/Stair Generator  t=SwitchTimesB  e=SwitchStatusB  Ts=0
  Switch2 : Switch  Criteria=u2 > Threshold  Threshold=0.5
  Switch3 : Switch  Criteria=u2 > Threshold  Threshold=0.5
  Switch4 : Switch  Criteria=u2 > Threshold  Threshold=0.5
  A : PMIOPort  Side=Left
  B : PMIOPort  Port=2  Side=Left
  C : PMIOPort  Port=3  Side=Left
  a : PMIOPort  Port=4  Side=Right
  b : PMIOPort  Port=5  Side=Right
  c : PMIOPort  Port=6  Side=Right
  wires:
  Switch2/1 -> Ideal Switch C/1
  Fault A2/1 -> Switch2/3
  Fault C1/1 -> Switch2/2
  Switch3/1 -> Ideal Switch B/1
  Fault A3/1 -> Switch3/3
  Fault C2/1 -> Switch3/2
  Fault A4/1 -> Switch4/3
  Fault C3/1 -> Switch4/2
  Switch4/1 -> Ideal Switch A/1
  Stair Generator B/1 -> Switch3/1
  Stair Generator A/1 -> Switch4/1
  Stair Generator C/1 -> Switch2/1
  connections:
  Ideal Switch B/LConn1 -- B/RConn1
  Ideal Switch A/LConn1 -- A/RConn1
  Ideal Switch C/LConn1 -- C/RConn1
  Ideal Switch A/RConn1 -- a/RConn1
  b/RConn1 -- Ideal Switch B/RConn1
  c/RConn1 -- Ideal Switch C/RConn1

== system SPGF_FSK_0000_R2019b/W35/Q/meas ==
  Add : Sum  Inputs=+++
  GainI : Gain
  GainI0 : Gain
  I A: : powerlib/Measurements/Current Measurement  PhasorSimulation=off  OutputType=Complex  PSBequivalent=0
  I B: : powerlib/Measurements/Current Measurement  PhasorSimulation=off  OutputType=Complex  PSBequivalent=0
  I C: : powerlib/Measurements/Current Measurement  PhasorSimulation=off  OutputType=Complex  PSBequivalent=0
  Mux : Mux  Inputs=3
  A : PMIOPort  Side=Left
  B : PMIOPort  Port=2  Side=Left
  C : PMIOPort  Port=3  Side=Left
  a : PMIOPort  Port=4  Side=Right
  b : PMIOPort  Port=5  Side=Right
  c : PMIOPort  Port=6  Side=Right
  tag scope: CT3I0_W35=global, CTIabc_W35=global
  wires:
  I A:/1 -> Mux/1, Add/1
  I B:/1 -> Mux/2, Add/2
  I C:/1 -> Mux/3, Add/3
  Add/1 -> GainI0/1
  GainI0/1 -> [CT3I0_W35]
  Mux/1 -> GainI/1
  GainI/1 -> [CTIabc_W35]
  connections:
  I C:/RConn1 -- c/RConn1
  I B:/RConn1 -- b/RConn1
  a/RConn1 -- I A:/RConn1
  I A:/LConn1 -- A/RConn1
  I C:/LConn1 -- C/RConn1
  I B:/LConn1 -- B/RConn1

== system SPGF_FSK_0000_R2019b/W35/Q/shunt ==
  A : PMIOPort  Side=Left
  B : PMIOPort  Port=2  Side=Left
  C : PMIOPort  Port=3  Side=Left
  a : PMIOPort  Port=4  Side=Right
  b : PMIOPort  Port=5  Side=Right
  c : PMIOPort  Port=6  Side=Right
  connections:
  C/RConn1 -- c/RConn1
  B/RConn1 -- b/RConn1
  A/RConn1 -- a/RConn1

== system SPGF_FSK_0000_R2019b/W41/Q/breaker ==
  Fault A2 : Constant  Value=InitialStatus(3)
  Fault A3 : Constant  Value=InitialStatus(2)
  Fault A4 : Constant  Value=InitialStatus(1)
  Fault C1 : Constant  Value=SwitchC
  Fault C2 : Constant  Value=SwitchB
  Fault C3 : Constant  Value=SwitchA
  Ideal Switch A : powerlib/Power Electronics/Ideal Switch  Ron=BreakerResistance  Lon=0  IC=InitialStatus(1)  Rs=SnubberResistance  Cs=SnubberCapacitance  Measurements=off
  Ideal Switch B : powerlib/Power Electronics/Ideal Switch  Ron=BreakerResistance  Lon=0  IC=InitialStatus(2)  Rs=SnubberResistance  Cs=SnubberCapacitance  Measurements=off
  Ideal Switch C : powerlib/Power Electronics/Ideal Switch  Ron=BreakerResistance  Lon=0  IC=InitialStatus(3)  Rs=SnubberResistance  Cs=SnubberCapacitance  Measurements=off
  Stair Generator A : powerlib_meascontrol/Pulse & Signal Generators/Stair Generator  t=SwitchTimesA  e=SwitchStatusA  Ts=0
  Stair Generator B : powerlib_meascontrol/Pulse & Signal Generators/Stair Generator  t=SwitchTimesB  e=SwitchStatusB  Ts=0
  Stair Generator C : powerlib_meascontrol/Pulse & Signal Generators/Stair Generator  t=SwitchTimesC  e=SwitchStatusC  Ts=0
  Switch2 : Switch  Criteria=u2 > Threshold  Threshold=0.5
  Switch3 : Switch  Criteria=u2 > Threshold  Threshold=0.5
  Switch4 : Switch  Criteria=u2 > Threshold  Threshold=0.5
  A : PMIOPort  Side=Left
  B : PMIOPort  Port=2  Side=Left
  C : PMIOPort  Port=3  Side=Left
  a : PMIOPort  Port=4  Side=Right
  b : PMIOPort  Port=5  Side=Right
  c : PMIOPort  Port=6  Side=Right
  wires:
  Switch2/1 -> Ideal Switch C/1
  Fault A2/1 -> Switch2/3
  Fault C1/1 -> Switch2/2
  Switch3/1 -> Ideal Switch B/1
  Fault A3/1 -> Switch3/3
  Fault C2/1 -> Switch3/2
  Fault A4/1 -> Switch4/3
  Fault C3/1 -> Switch4/2
  Switch4/1 -> Ideal Switch A/1
  Stair Generator B/1 -> Switch3/1
  Stair Generator A/1 -> Switch4/1
  Stair Generator C/1 -> Switch2/1
  connections:
  Ideal Switch B/LConn1 -- B/RConn1
  Ideal Switch A/LConn1 -- A/RConn1
  Ideal Switch C/LConn1 -- C/RConn1
  Ideal Switch A/RConn1 -- a/RConn1
  b/RConn1 -- Ideal Switch B/RConn1
  c/RConn1 -- Ideal Switch C/RConn1

== system SPGF_FSK_0000_R2019b/W41/Q/meas ==
  Add : Sum  Inputs=+++
  GainI : Gain
  GainI0 : Gain
  I A: : powerlib/Measurements/Current Measurement  PhasorSimulation=off  OutputType=Complex  PSBequivalent=0
  I B: : powerlib/Measurements/Current Measurement  PhasorSimulation=off  OutputType=Complex  PSBequivalent=0
  I C: : powerlib/Measurements/Current Measurement  PhasorSimulation=off  OutputType=Complex  PSBequivalent=0
  Mux : Mux  Inputs=3
  A : PMIOPort  Side=Left
  B : PMIOPort  Port=2  Side=Left
  C : PMIOPort  Port=3  Side=Left
  a : PMIOPort  Port=4  Side=Right
  b : PMIOPort  Port=5  Side=Right
  c : PMIOPort  Port=6  Side=Right
  tag scope: CT3I0_W41=global, CTIabc_W41=global
  wires:
  I A:/1 -> Mux/1, Add/1
  I B:/1 -> Mux/2, Add/2
  I C:/1 -> Mux/3, Add/3
  Add/1 -> GainI0/1
  GainI0/1 -> [CT3I0_W41]
  Mux/1 -> GainI/1
  GainI/1 -> [CTIabc_W41]
  connections:
  I C:/RConn1 -- c/RConn1
  I B:/RConn1 -- b/RConn1
  a/RConn1 -- I A:/RConn1
  I A:/LConn1 -- A/RConn1
  I C:/LConn1 -- C/RConn1
  I B:/LConn1 -- B/RConn1

== system SPGF_FSK_0000_R2019b/W41/Q/shunt ==
  A : PMIOPort  Side=Left
  B : PMIOPort  Port=2  Side=Left
  C : PMIOPort  Port=3  Side=Left
  a : PMIOPort  Port=4  Side=Right
  b : PMIOPort  Port=5  Side=Right
  c : PMIOPort  Port=6  Side=Right
  connections:
  C/RConn1 -- c/RConn1
  B/RConn1 -- b/RConn1
  A/RConn1 -- a/RConn1

== system SPGF_FSK_0000_R2019b/W42/Q/breaker ==
  Fault A2 : Constant  Value=InitialStatus(3)
  Fault A3 : Constant  Value=InitialStatus(2)
  Fault A4 : Constant  Value=InitialStatus(1)
  Fault C1 : Constant  Value=SwitchC
  Fault C2 : Constant  Value=SwitchB
  Fault C3 : Constant  Value=SwitchA
  Ideal Switch A : powerlib/Power Electronics/Ideal Switch  Ron=BreakerResistance  Lon=0  IC=InitialStatus(1)  Rs=SnubberResistance  Cs=SnubberCapacitance  Measurements=off
  Ideal Switch B : powerlib/Power Electronics/Ideal Switch  Ron=BreakerResistance  Lon=0  IC=InitialStatus(2)  Rs=SnubberResistance  Cs=SnubberCapacitance  Measurements=off
  Ideal Switch C : powerlib/Power Electronics/Ideal Switch  Ron=BreakerResistance  Lon=0  IC=InitialStatus(3)  Rs=SnubberResistance  Cs=SnubberCapacitance  Measurements=off
  Stair Generator A : powerlib_meascontrol/Pulse & Signal Generators/Stair Generator  t=SwitchTimesA  e=SwitchStatusA  Ts=0
  Stair Generator B : powerlib_meascontrol/Pulse & Signal Generators/Stair Generator  t=SwitchTimesB  e=SwitchStatusB  Ts=0
  Stair Generator C : powerlib_meascontrol/Pulse & Signal Generators/Stair Generator  t=SwitchTimesB  e=SwitchStatusB  Ts=0
  Switch2 : Switch  Criteria=u2 > Threshold  Threshold=0.5
  Switch3 : Switch  Criteria=u2 > Threshold  Threshold=0.5
  Switch4 : Switch  Criteria=u2 > Threshold  Threshold=0.5
  A : PMIOPort  Side=Left
  B : PMIOPort  Port=2  Side=Left
  C : PMIOPort  Port=3  Side=Left
  a : PMIOPort  Port=4  Side=Right
  b : PMIOPort  Port=5  Side=Right
  c : PMIOPort  Port=6  Side=Right
  wires:
  Switch2/1 -> Ideal Switch C/1
  Fault A2/1 -> Switch2/3
  Fault C1/1 -> Switch2/2
  Switch3/1 -> Ideal Switch B/1
  Fault A3/1 -> Switch3/3
  Fault C2/1 -> Switch3/2
  Fault A4/1 -> Switch4/3
  Fault C3/1 -> Switch4/2
  Switch4/1 -> Ideal Switch A/1
  Stair Generator B/1 -> Switch3/1
  Stair Generator A/1 -> Switch4/1
  Stair Generator C/1 -> Switch2/1
  connections:
  Ideal Switch B/LConn1 -- B/RConn1
  Ideal Switch A/LConn1 -- A/RConn1
  Ideal Switch C/LConn1 -- C/RConn1
  Ideal Switch A/RConn1 -- a/RConn1
  b/RConn1 -- Ideal Switch B/RConn1
  c/RConn1 -- Ideal Switch C/RConn1

== system SPGF_FSK_0000_R2019b/W42/Q/meas ==
  Add : Sum  Inputs=+++
  GainI : Gain
  GainI0 : Gain
  I A: : powerlib/Measurements/Current Measurement  PhasorSimulation=off  OutputType=Complex  PSBequivalent=0
  I B: : powerlib/Measurements/Current Measurement  PhasorSimulation=off  OutputType=Complex  PSBequivalent=0
  I C: : powerlib/Measurements/Current Measurement  PhasorSimulation=off  OutputType=Complex  PSBequivalent=0
  Mux : Mux  Inputs=3
  A : PMIOPort  Side=Left
  B : PMIOPort  Port=2  Side=Left
  C : PMIOPort  Port=3  Side=Left
  a : PMIOPort  Port=4  Side=Right
  b : PMIOPort  Port=5  Side=Right
  c : PMIOPort  Port=6  Side=Right
  tag scope: CT3I0_W42=global, CTIabc_W42=global
  wires:
  I A:/1 -> Mux/1, Add/1
  I B:/1 -> Mux/2, Add/2
  I C:/1 -> Mux/3, Add/3
  Add/1 -> GainI0/1
  GainI0/1 -> [CT3I0_W42]
  Mux/1 -> GainI/1
  GainI/1 -> [CTIabc_W42]
  connections:
  I C:/RConn1 -- c/RConn1
  I B:/RConn1 -- b/RConn1
  a/RConn1 -- I A:/RConn1
  I A:/LConn1 -- A/RConn1
  I C:/LConn1 -- C/RConn1
  I B:/LConn1 -- B/RConn1

== system SPGF_FSK_0000_R2019b/W42/Q/shunt ==
  A : PMIOPort  Side=Left
  B : PMIOPort  Port=2  Side=Left
  C : PMIOPort  Port=3  Side=Left
  a : PMIOPort  Port=4  Side=Right
  b : PMIOPort  Port=5  Side=Right
  c : PMIOPort  Port=6  Side=Right
  connections:
  C/RConn1 -- c/RConn1
  B/RConn1 -- b/RConn1
  A/RConn1 -- a/RConn1

== system SPGF_FSK_0000_R2019b/W43/Q/breaker ==
  Fault A2 : Constant  Value=InitialStatus(3)
  Fault A3 : Constant  Value=InitialStatus(2)
  Fault A4 : Constant  Value=InitialStatus(1)
  Fault C1 : Constant  Value=SwitchC
  Fault C2 : Constant  Value=SwitchB
  Fault C3 : Constant  Value=SwitchA
  Ideal Switch A : powerlib/Power Electronics/Ideal Switch  Ron=BreakerResistance  Lon=0  IC=InitialStatus(1)  Rs=SnubberResistance  Cs=SnubberCapacitance  Measurements=off
  Ideal Switch B : powerlib/Power Electronics/Ideal Switch  Ron=BreakerResistance  Lon=0  IC=InitialStatus(2)  Rs=SnubberResistance  Cs=SnubberCapacitance  Measurements=off
  Ideal Switch C : powerlib/Power Electronics/Ideal Switch  Ron=BreakerResistance  Lon=0  IC=InitialStatus(3)  Rs=SnubberResistance  Cs=SnubberCapacitance  Measurements=off
  Stair Generator A : powerlib_meascontrol/Pulse & Signal Generators/Stair Generator  t=SwitchTimesA  e=SwitchStatusA  Ts=0
  Stair Generator B : powerlib_meascontrol/Pulse & Signal Generators/Stair Generator  t=SwitchTimesB  e=SwitchStatusB  Ts=0
  Stair Generator C : powerlib_meascontrol/Pulse & Signal Generators/Stair Generator  t=SwitchTimesB  e=SwitchStatusB  Ts=0
  Switch2 : Switch  Criteria=u2 > Threshold  Threshold=0.5
  Switch3 : Switch  Criteria=u2 > Threshold  Threshold=0.5
  Switch4 : Switch  Criteria=u2 > Threshold  Threshold=0.5
  A : PMIOPort  Side=Left
  B : PMIOPort  Port=2  Side=Left
  C : PMIOPort  Port=3  Side=Left
  a : PMIOPort  Port=4  Side=Right
  b : PMIOPort  Port=5  Side=Right
  c : PMIOPort  Port=6  Side=Right
  wires:
  Switch2/1 -> Ideal Switch C/1
  Fault A2/1 -> Switch2/3
  Fault C1/1 -> Switch2/2
  Switch3/1 -> Ideal Switch B/1
  Fault A3/1 -> Switch3/3
  Fault C2/1 -> Switch3/2
  Fault A4/1 -> Switch4/3
  Fault C3/1 -> Switch4/2
  Switch4/1 -> Ideal Switch A/1
  Stair Generator B/1 -> Switch3/1
  Stair Generator A/1 -> Switch4/1
  Stair Generator C/1 -> Switch2/1
  connections:
  Ideal Switch B/LConn1 -- B/RConn1
  Ideal Switch A/LConn1 -- A/RConn1
  Ideal Switch C/LConn1 -- C/RConn1
  Ideal Switch A/RConn1 -- a/RConn1
  b/RConn1 -- Ideal Switch B/RConn1
  c/RConn1 -- Ideal Switch C/RConn1

== system SPGF_FSK_0000_R2019b/W43/Q/meas ==
  Add : Sum  Inputs=+++
  GainI : Gain
  GainI0 : Gain
  I A: : powerlib/Measurements/Current Measurement  PhasorSimulation=off  OutputType=Complex  PSBequivalent=0
  I B: : powerlib/Measurements/Current Measurement  PhasorSimulation=off  OutputType=Complex  PSBequivalent=0
  I C: : powerlib/Measurements/Current Measurement  PhasorSimulation=off  OutputType=Complex  PSBequivalent=0
  Mux : Mux  Inputs=3
  A : PMIOPort  Side=Left
  B : PMIOPort  Port=2  Side=Left
  C : PMIOPort  Port=3  Side=Left
  a : PMIOPort  Port=4  Side=Right
  b : PMIOPort  Port=5  Side=Right
  c : PMIOPort  Port=6  Side=Right
  tag scope: CT3I0_W43=global, CTIabc_W43=global
  wires:
  I A:/1 -> Mux/1, Add/1
  I B:/1 -> Mux/2, Add/2
  I C:/1 -> Mux/3, Add/3
  Add/1 -> GainI0/1
  GainI0/1 -> [CT3I0_W43]
  Mux/1 -> GainI/1
  GainI/1 -> [CTIabc_W43]
  connections:
  I C:/RConn1 -- c/RConn1
  I B:/RConn1 -- b/RConn1
  a/RConn1 -- I A:/RConn1
  I A:/LConn1 -- A/RConn1
  I C:/LConn1 -- C/RConn1
  I B:/LConn1 -- B/RConn1

== system SPGF_FSK_0000_R2019b/W43/Q/shunt ==
  A : PMIOPort  Side=Left
  B : PMIOPort  Port=2  Side=Left
  C : PMIOPort  Port=3  Side=Left
  a : PMIOPort  Port=4  Side=Right
  b : PMIOPort  Port=5  Side=Right
  c : PMIOPort  Port=6  Side=Right
  connections:
  C/RConn1 -- c/RConn1
  B/RConn1 -- b/RConn1
  A/RConn1 -- a/RConn1
